simulink model "fixed_2"  (Simulink 2.20)
settings: Solver=ode45  StartTime=0.0  StopTime=10.0  RelTol=1e-3  AbsTol=1e-6
settings Model: OutputOption=SpecifiedOutputTimes  OutputTimes=[0:0.01:10]  LimitMaxRows=on  ConsistencyChecking=off  RTWPlaceOutputsASAP=off

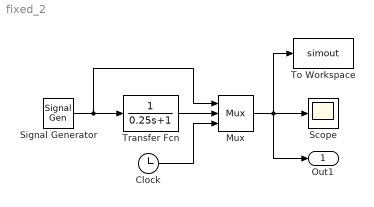
== system fixed_2 ==
  Clock : Clock
  Mux : Mux  Inputs=3
  Scope : Scope
      settings: TickLabels=on  TimeRange=auto  YMin=-5  YMax=5  SaveToWorkspace=off  SaveName=ScopeData
  Signal Generator : SignalGenerator  WaveForm=square  Amplitude=1  Frequency=0.5  Units=Hertz
  To Workspace : ToWorkspace  VariableName=simout  SampleTime=-1
  Transfer Fcn : TransferFcn  Numerator=[1]  Denominator=[0.25 1]
  Out1 : Outport  Port=1
  wires:
  Transfer Fcn/1 -> Mux/2
  Signal Generator/1 -> Transfer Fcn/1, Mux/1
  Mux/1 -> Out1/1, Scope/1, To Workspace/1
  Clock/1 -> Mux/3
